simulink model "RTR_1st"  (R2020a)
settings: Solver=ode45  StartTime=0.0  StopTime=T  RelTol=1e-8
values from neighbouring files (symbols this model uses):
  g = 9.81    [TestingIkRTR.m]    (also in TestingScript.m; TestingScriptRTR.m)
  Kd1 = Kp1/10    (= 100)    [TestingIkRTR.m]    (also in TestingScript.m; TestingScriptRTR.m)
  Kp1 = 1000    [TestingIkRTR.m]    (also in TestingScript.m; TestingScriptRTR.m)
  l2 = 0.3    [TestingIkRTR.m]    (also in TestingScriptRTR.m)
  l3 = 0.2    [TestingIkRTR.m]    (also in TestingScriptRTR.m)
  m2 = 20    [TestingIkRTR.m]    (also in TestingScriptRTR.m)
  m3 = 20    [TestingIkRTR.m]    (also in TestingScriptRTR.m)
settings Model: Creator=ja  LastModifiedBy=ja

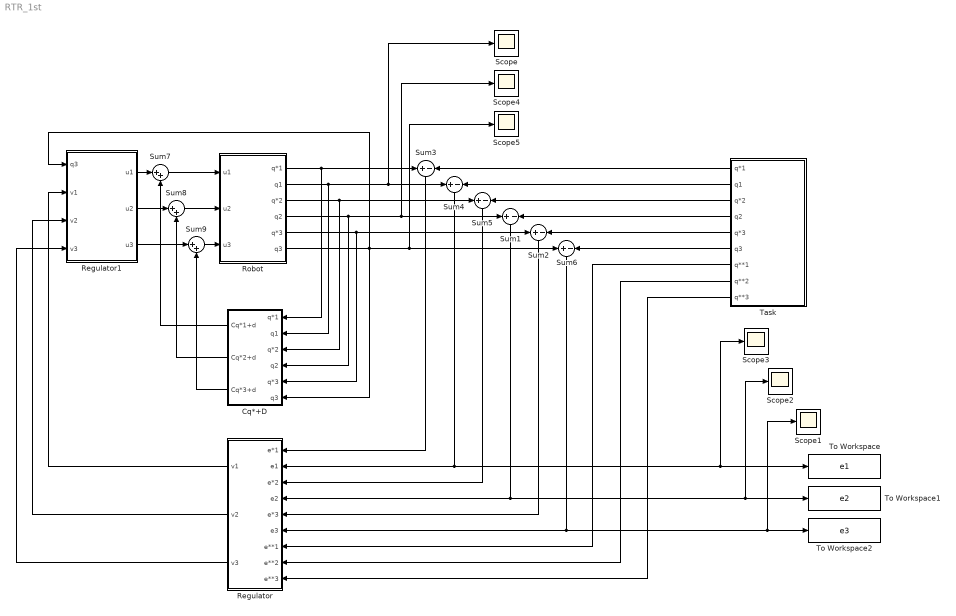
== system RTR_1st ==
  Cq*+D : Subsystem
  Regulator : Subsystem
  Regulator1 : Subsystem
  Robot : Subsystem
  Scope{,1..5} (6 alike) : Scope
  Sum{1..6} (6 alike) : Sum  Inputs=+-
  Sum7 : Sum  Inputs=|++
  Sum8 : Sum  Inputs=|++
  Sum9 : Sum  Inputs=|++
  Task : Subsystem
  To Workspace : ToWorkspace  VariableName=e1  SampleTime=-1
  To Workspace1 : ToWorkspace  VariableName=e2  SampleTime=-1
  To Workspace2 : ToWorkspace  VariableName=e3  SampleTime=-1
  wires:
  Robot/1(q*1) -> Cq*+D/1(q*1), Sum3/1
  Task/1(q*1) -> Sum3/2
  Robot/2(q1) -> Cq*+D/2(q1), Scope/1, Sum4/1
  Task/2(q1) -> Sum4/2
  Task/3(q*2) -> Sum5/2
  Robot/3(q*2) -> Cq*+D/3(q*2), Sum5/1
  Task/4(q2) -> Sum1/2
  Robot/4(q2) -> Cq*+D/4(q2), Scope4/1, Sum1/1
  Task/5(q*3) -> Sum2/2
  Robot/5(q*3) -> Cq*+D/5(q*3), Sum2/1
  Task/6(q3) -> Sum6/2
  Robot/6(q3) -> Regulator1/1(q3), Cq*+D/6(q3), Scope5/1, Sum6/1
  Sum3/1 -> Regulator/1(e*1)
  Sum4/1 -> Scope3/1, To Workspace/1, Regulator/2(e1)
  Sum5/1 -> Regulator/3(e*2)
  Sum1/1 -> Scope2/1, To Workspace1/1, Regulator/4(e2)
  Sum2/1 -> Regulator/5(e*3)
  Sum6/1 -> Scope1/1, To Workspace2/1, Regulator/6(e3)
  Regulator/1(" v1") -> Regulator1/2(v1)
  Regulator/2(v2) -> Regulator1/3(v2)
  Regulator/3(v3) -> Regulator1/4(v3)
  Sum7/1 -> Robot/1(u1)
  Regulator1/1(" u1") -> Sum7/1
  Regulator1/2(u2) -> Sum8/1
  Sum8/1 -> Robot/2(u2)
  Regulator1/3(u3) -> Sum9/1
  Sum9/1 -> Robot/3(u3)
  Cq*+D/1(" Cq*1+d") -> Sum7/2
  Cq*+D/2(Cq*2+d) -> Sum8/2
  Cq*+D/3(Cq*3+d) -> Sum9/2
  Task/7(q**1) -> Regulator/7(e**1)
  Task/8(q**2) -> Regulator/8(e**2)
  Task/9(q**3) -> Regulator/9(e**3)

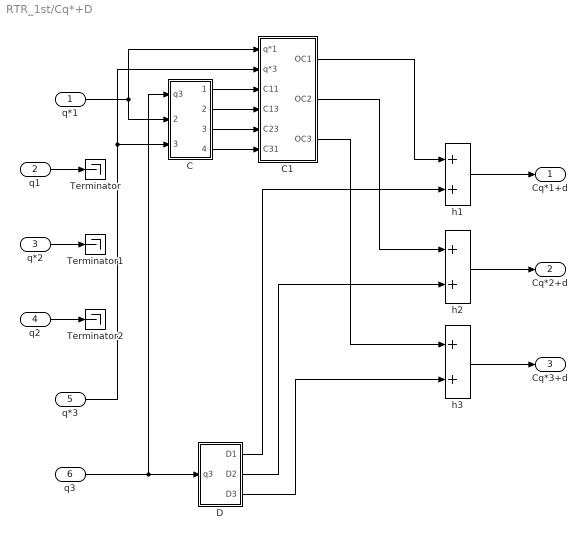
== system RTR_1st/Cq*+D ==
  q*1 : Inport
  q1 : Inport  Port=2
  q*2 : Inport  Port=3
  q2 : Inport  Port=4
  q*3 : Inport  Port=5
  q3 : Inport  Port=6
  C : Subsystem
  C1 : Subsystem
  D : Subsystem
  Terminator : Terminator
  Terminator1 : Terminator
  Terminator2 : Terminator
  h1 : Sum
  h2 : Sum
  h3 : Sum
  " Cq*1+d" : Outport
  Cq*2+d : Outport  Port=2
  Cq*3+d : Outport  Port=3
  wires:
  D/1(D1) -> h1/2
  D/2(D2) -> h2/2
  C1/2(OC2) -> h2/1
  D/3(D3) -> h3/2
  C/2(C13) -> C1/4(C13)
  C/1(C11) -> C1/3(C11)
  C/3(C23) -> C1/5(C23)
  C1/1(OC1) -> h1/1
  C/4(C31) -> C1/6(C31)
  C1/3(OC3) -> h3/1
  q3/1 -> C/1(q3), D/1(q3)
  h1/1 -> " Cq*1+d"/1
  h2/1 -> Cq*2+d/1
  h3/1 -> Cq*3+d/1
  q*1/1 -> C1/1(q*1), C/2(q*1)
  q*3/1 -> C/3(q*3), C1/2(q*3)
  q1/1 -> Terminator/1
  q*2/1 -> Terminator1/1
  q2/1 -> Terminator2/1

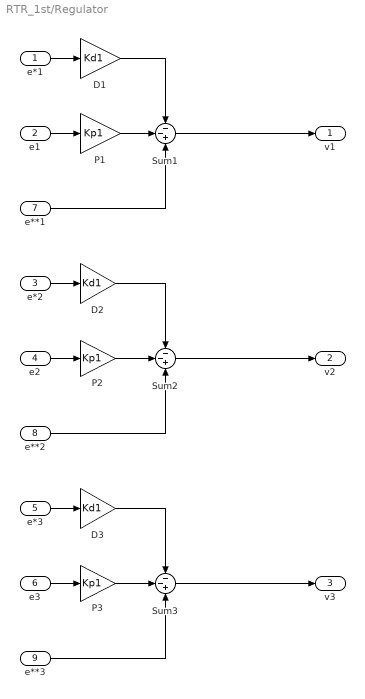
== system RTR_1st/Regulator ==
  e*1 : Inport
  e1 : Inport  Port=2
  e*2 : Inport  Port=3
  e2 : Inport  Port=4
  e*3 : Inport  Port=5
  e3 : Inport  Port=6
  e**1 : Inport  Port=7
  e**2 : Inport  Port=8
  e**3 : Inport  Port=9
  D1 : Gain  Gain=Kd1
  D2 : Gain  Gain=Kd1
  D3 : Gain  Gain=Kd1
  P1 : Gain  Gain=Kp1
  P2 : Gain  Gain=Kp1
  P3 : Gain  Gain=Kp1
  Sum1 : Sum  Inputs=--+
  Sum2 : Sum  Inputs=--+
  Sum3 : Sum  Inputs=--+
  " v1" : Outport
  v2 : Outport  Port=2
  v3 : Outport  Port=3
  wires:
  e2/1 -> P2/1
  Sum2/1 -> v2/1
  e*2/1 -> D2/1
  e1/1 -> P1/1
  Sum1/1 -> " v1"/1
  e*1/1 -> D1/1
  D1/1 -> Sum1/1
  P1/1 -> Sum1/2
  D2/1 -> Sum2/1
  P2/1 -> Sum2/2
  e*3/1 -> D3/1
  Sum3/1 -> v3/1
  P3/1 -> Sum3/2
  D3/1 -> Sum3/1
  e3/1 -> P3/1
  e**1/1 -> Sum1/3
  e**2/1 -> Sum2/3
  e**3/1 -> Sum3/3

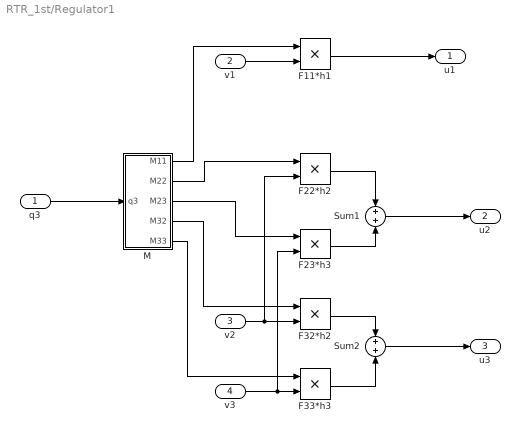
== system RTR_1st/Regulator1 ==
  q3 : Inport
  v1 : Inport  Port=2
  v2 : Inport  Port=3
  v3 : Inport  Port=4
  F11*h1 : Product
  F22*h2 : Product
  F23*h3 : Product
  F32*h2 : Product
  F33*h3 : Product
  M : Subsystem
  Sum1 : Sum
  Sum2 : Sum
  " u1" : Outport
  u2 : Outport  Port=2
  u3 : Outport  Port=3
  wires:
  q3/1 -> M/1(q3)
  F23*h3/1 -> Sum1/2
  F33*h3/1 -> Sum2/2
  F22*h2/1 -> Sum1/1
  F32*h2/1 -> Sum2/1
  v3/1 -> F23*h3/2, F33*h3/2
  v2/1 -> F22*h2/2, F32*h2/2
  v1/1 -> F11*h1/2
  M/1(M11) -> F11*h1/1
  M/2(M22) -> F22*h2/1
  M/3(M23) -> F23*h3/1
  M/4(M32) -> F32*h2/1
  M/5(M33) -> F33*h3/1
  F11*h1/1 -> " u1"/1
  Sum1/1 -> u2/1
  Sum2/1 -> u3/1

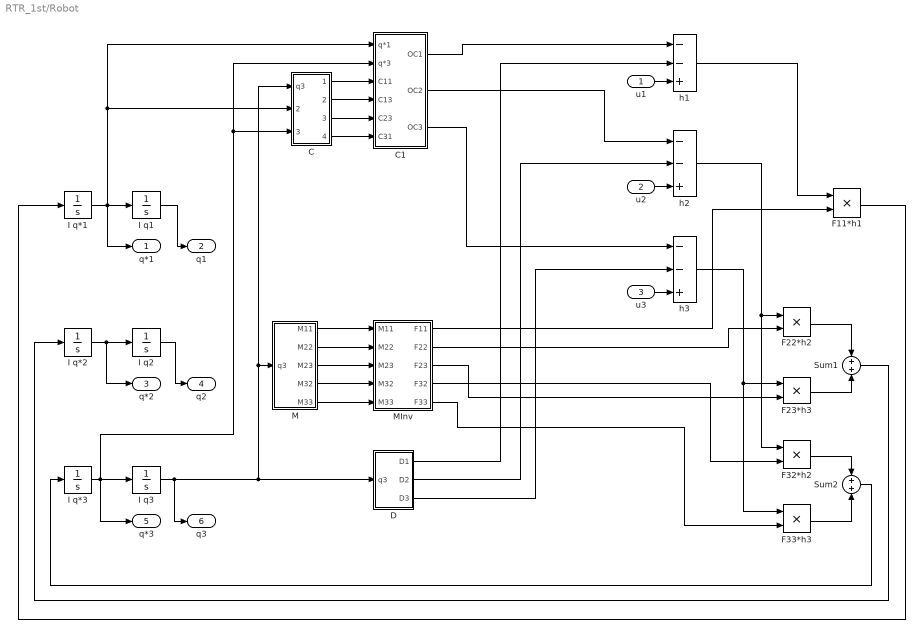
== system RTR_1st/Robot ==
  u1 : Inport
  u2 : Inport  Port=2
  u3 : Inport  Port=3
  C : Subsystem
  C1 : Subsystem
  D : Subsystem
  F11*h1 : Product
  F22*h2 : Product
  F23*h3 : Product
  F32*h2 : Product
  F33*h3 : Product
  I q*1 : Integrator
  I q*2 : Integrator
  I q*3 : Integrator
  I q1 : Integrator
  I q2 : Integrator
  I q3 : Integrator
  M : Subsystem
  MInv : MATLAB Function  TreatAsAtomicUnit=on
  Sum1 : Sum
  Sum2 : Sum
  h1 : Sum  Inputs=--+
  h2 : Sum  Inputs=--+
  h3 : Sum  Inputs=--+
  q*1 : Outport
  q1 : Outport  Port=2
  q*2 : Outport  Port=3
  q2 : Outport  Port=4
  q*3 : Outport  Port=5
  q3 : Outport  Port=6
  wires:
  I q2/1 -> q2/1
  F11*h1/1 -> I q*1/1
  I q*1/1 -> q*1/1, C1/1(q*1), C/2(q*1), I q1/1
  Sum1/1 -> I q*2/1
  I q1/1 -> q1/1
  F23*h3/1 -> Sum1/2
  I q*2/1 -> q*2/1, I q2/1
  F22*h2/1 -> Sum1/1
  u2/1 -> h2/3
  C/1(C11) -> C1/3(C11)
  C/2(C13) -> C1/4(C13)
  C/3(C23) -> C1/5(C23)
  C/4(C31) -> C1/6(C31)
  C1/1(OC1) -> h1/1
  F32*h2/1 -> Sum2/1
  F33*h3/1 -> Sum2/2
  Sum2/1 -> I q*3/1
  I q*3/1 -> C1/2(q*3), C/3(q*3), I q3/1, q*3/1
  I q3/1 -> q3/1, C/1(q3), M/1(q3), D/1(q3)
  u3/1 -> h3/3
  D/3(D3) -> h3/2
  D/2(D2) -> h2/2
  C1/2(OC2) -> h2/1
  C1/3(OC3) -> h3/1
  h2/1 -> F32*h2/1, F22*h2/1
  h3/1 -> F33*h3/1, F23*h3/1
  MInv/2(F22) -> F22*h2/2
  MInv/3(F23) -> F23*h3/2
  MInv/4(F32) -> F32*h2/2
  MInv/5(F33) -> F33*h3/2
  h1/1 -> F11*h1/1
  MInv/1(F11) -> F11*h1/2
  u1/1 -> h1/3
  D/1(D1) -> h1/2
  M/1(M11) -> MInv/1(M11)
  M/2(M22) -> MInv/2(M22)
  M/3(M23) -> MInv/3(M23)
  M/4(M32) -> MInv/4(M32)
  M/5(M33) -> MInv/5(M33)

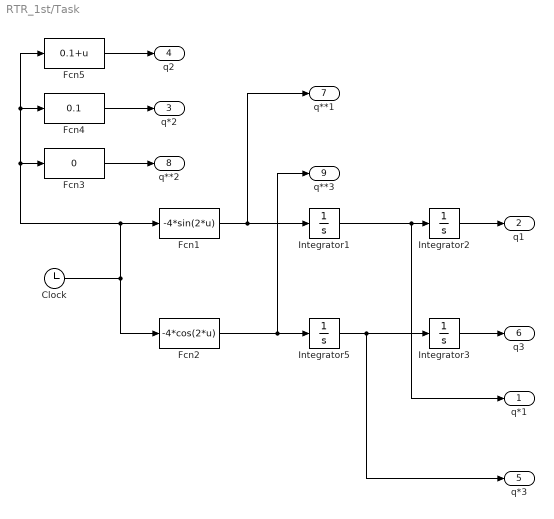
== system RTR_1st/Task ==
  Clock : Clock
  Fcn1 : Fcn  Expr=-4*sin(2*u)
  Fcn2 : Fcn  Expr=-4*cos(2*u)
  Fcn3 : Fcn  Expr=0
  Fcn4 : Fcn  Expr=0.1
  Fcn5 : Fcn  Expr=0.1+u
  Integrator1 : Integrator  InitialCondition=2
  Integrator2 : Integrator
  Integrator3 : Integrator  InitialCondition=1
  Integrator5 : Integrator
  q*1 : Outport
  q1 : Outport  Port=2
  q*2 : Outport  Port=3
  q2 : Outport  Port=4
  q*3 : Outport  Port=5
  q3 : Outport  Port=6
  q**1 : Outport  Port=7
  q**2 : Outport  Port=8
  q**3 : Outport  Port=9
  wires:
  Integrator2/1 -> q1/1
  Integrator3/1 -> q3/1
  Integrator1/1 -> q*1/1, Integrator2/1
  Integrator5/1 -> q*3/1, Integrator3/1
  Fcn1/1 -> Integrator1/1, q**1/1
  Fcn2/1 -> q**3/1, Integrator5/1
  Fcn3/1 -> q**2/1
  Fcn4/1 -> q*2/1
  Fcn5/1 -> q2/1
  Clock/1 -> Fcn5/1, Fcn4/1, Fcn3/1, Fcn1/1, Fcn2/1

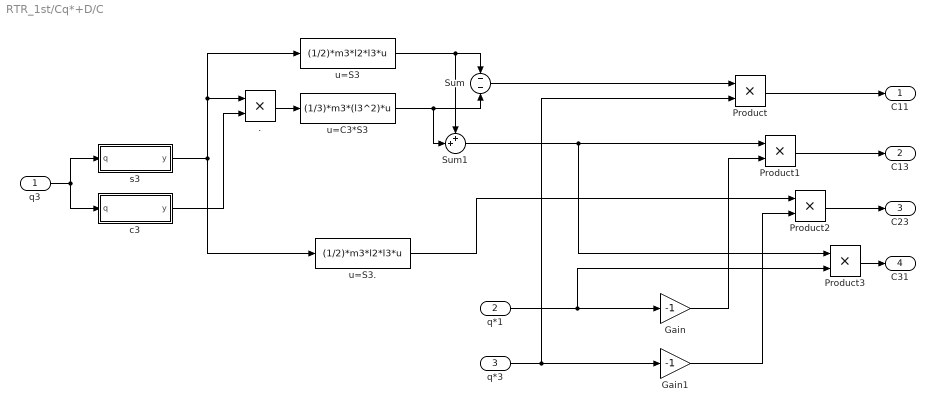
== system RTR_1st/Cq*+D/C ==
  q3 : Inport
  q*1 : Inport  Port=2
  q*3 : Inport  Port=3
  . : Product
  Gain : Gain  Gain=-1
  Gain1 : Gain  Gain=-1
  Product{,1..3} (4 alike) : Product
  Sum : Sum  Inputs=--
  Sum1 : Sum  Inputs=++|
  c3 : MATLAB Function  TreatAsAtomicUnit=on
  s3 : MATLAB Function  TreatAsAtomicUnit=on
  u=C3*S3 : Fcn  Expr=(1/3)*m3*(l3^2)*u
  u=S3 : Fcn  Expr=(1/2)*m3*l2*l3*u
  u=S3. : Fcn  Expr=(1/2)*m3*l2*l3*u
  C11 : Outport
  C13 : Outport  Port=2
  C23 : Outport  Port=3
  C31 : Outport  Port=4
  wires:
  q3/1 -> s3/1(q), c3/1(q)
  c3/1(y) -> ./2
  s3/1(y) -> u=S3./1, ./1, u=S3/1
  ./1 -> u=C3*S3/1
  u=C3*S3/1 -> Sum1/2, Sum/2
  u=S3/1 -> Sum1/1, Sum/1
  Gain1/1 -> Product2/2
  Product/1 -> C11/1
  Product2/1 -> C23/1
  Product1/1 -> C13/1
  Sum/1 -> Product/1
  q*1/1 -> Gain/1, Product3/2
  q*3/1 -> Gain1/1, Product/2
  Product3/1 -> C31/1
  Gain/1 -> Product1/2
  Sum1/1 -> Product1/1, Product3/1
  u=S3./1 -> Product2/1

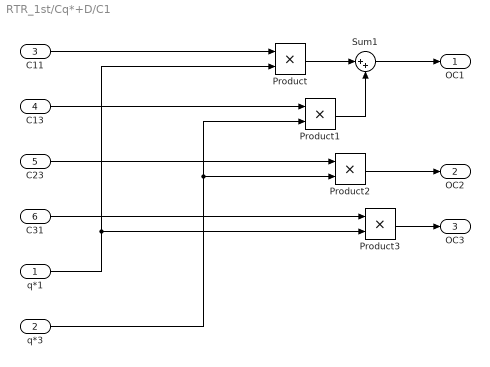
== system RTR_1st/Cq*+D/C1 ==
  q*1 : Inport
  q*3 : Inport  Port=2
  C11 : Inport  Port=3
  C13 : Inport  Port=4
  C23 : Inport  Port=5
  C31 : Inport  Port=6
  Product{,1..3} (4 alike) : Product
  Sum1 : Sum  Inputs=|++
  OC1 : Outport
  OC2 : Outport  Port=2
  OC3 : Outport  Port=3
  wires:
  C11/1 -> Product/1
  C13/1 -> Product1/1
  C23/1 -> Product2/1
  C31/1 -> Product3/1
  Product3/1 -> OC3/1
  Product2/1 -> OC2/1
  q*1/1 -> Product3/2, Product/2
  q*3/1 -> Product2/2, Product1/2
  Product/1 -> Sum1/1
  Sum1/1 -> OC1/1
  Product1/1 -> Sum1/2

== system RTR_1st/Cq*+D/D ==
  q3 : Inport
  . : Fcn  Expr=1/2*m3*l3*u
  Constant : Constant  Value=g
  Constant1 : Constant  Value=m3
  Constant2 : Constant  Value=m2
  Constant3 : Constant  Value=0
  Product : Product
  Product1 : Product
  Sum : Sum
  c3 : MATLAB Function  TreatAsAtomicUnit=on
  D1 : Outport
  D2 : Outport  Port=2
  D3 : Outport  Port=3
  wires:
  c3/1(y) -> ./1
  Sum/1 -> Product/1
  Constant/1 -> Product/2, Product1/1
  ./1 -> Product1/2
  Constant2/1 -> Sum/2
  Constant1/1 -> Sum/1
  q3/1 -> c3/1(q)
  Product/1 -> D2/1
  Product1/1 -> D3/1
  Constant3/1 -> D1/1

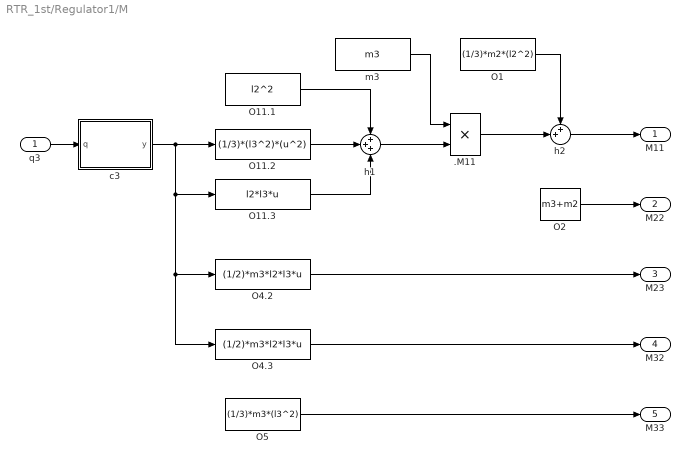
== system RTR_1st/Regulator1/M ==
  q3 : Inport
  .M11 : Product
  O1 : Constant  Value=(1/3)*m2*(l2^2)
  O11.1 : Constant  Value=l2^2
  O11.2 : Fcn  Expr=(1/3)*(l3^2)*(u^2)
  O11.3 : Fcn  Expr=l2*l3*u
  O2 : Constant  Value=m3+m2
  O4.2 : Fcn  Expr=(1/2)*m3*l2*l3*u
  O4.3 : Fcn  Expr=(1/2)*m3*l2*l3*u
  O5 : Constant  Value=(1/3)*m3*(l3^2)
  c3 : MATLAB Function  TreatAsAtomicUnit=on
  h1 : Sum  Inputs=+++
  h2 : Sum  Inputs=++|
  m3 : Constant  Value=m3
  M11 : Outport
  M22 : Outport  Port=2
  M23 : Outport  Port=3
  M32 : Outport  Port=4
  M33 : Outport  Port=5
  wires:
  O1/1 -> h2/1
  O11.3/1 -> h1/3
  m3/1 -> .M11/1
  h1/1 -> .M11/2
  .M11/1 -> h2/2
  O11.1/1 -> h1/1
  O11.2/1 -> h1/2
  h2/1 -> M11/1
  O2/1 -> M22/1
  O4.2/1 -> M23/1
  c3/1(y) -> O11.2/1, O4.3/1, O4.2/1, O11.3/1
  q3/1 -> c3/1(q)
  O5/1 -> M33/1
  O4.3/1 -> M32/1

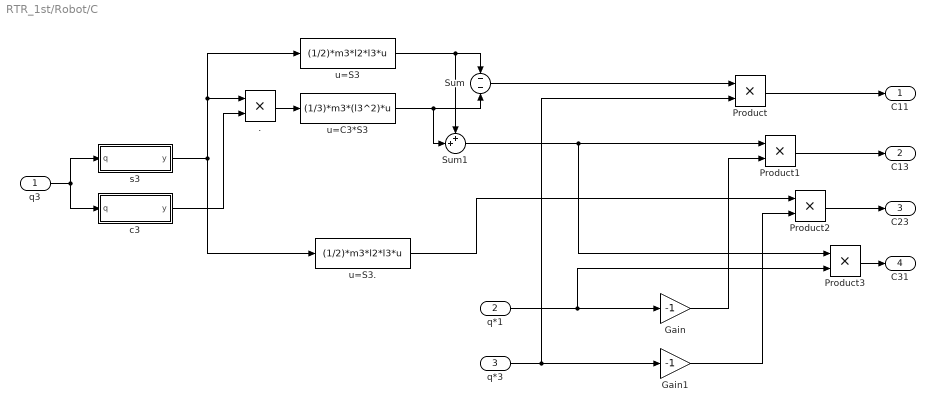
== system RTR_1st/Robot/C ==
  q3 : Inport
  q*1 : Inport  Port=2
  q*3 : Inport  Port=3
  . : Product
  Gain : Gain  Gain=-1
  Gain1 : Gain  Gain=-1
  Product{,1..3} (4 alike) : Product
  Sum : Sum  Inputs=--
  Sum1 : Sum  Inputs=++|
  c3 : MATLAB Function  TreatAsAtomicUnit=on
  s3 : MATLAB Function  TreatAsAtomicUnit=on
  u=C3*S3 : Fcn  Expr=(1/3)*m3*(l3^2)*u
  u=S3 : Fcn  Expr=(1/2)*m3*l2*l3*u
  u=S3. : Fcn  Expr=(1/2)*m3*l2*l3*u
  C11 : Outport
  C13 : Outport  Port=2
  C23 : Outport  Port=3
  C31 : Outport  Port=4
  wires:
  q3/1 -> s3/1(q), c3/1(q)
  c3/1(y) -> ./2
  s3/1(y) -> u=S3./1, ./1, u=S3/1
  ./1 -> u=C3*S3/1
  u=C3*S3/1 -> Sum1/2, Sum/2
  u=S3/1 -> Sum1/1, Sum/1
  Gain1/1 -> Product2/2
  Product/1 -> C11/1
  Product2/1 -> C23/1
  Product1/1 -> C13/1
  Sum/1 -> Product/1
  q*1/1 -> Gain/1, Product3/2
  q*3/1 -> Gain1/1, Product/2
  Product3/1 -> C31/1
  Gain/1 -> Product1/2
  Sum1/1 -> Product1/1, Product3/1
  u=S3./1 -> Product2/1

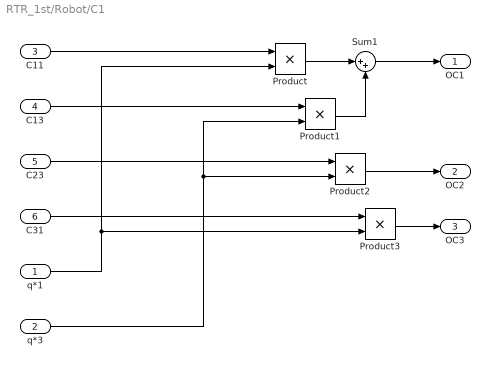
== system RTR_1st/Robot/C1 ==
  q*1 : Inport
  q*3 : Inport  Port=2
  C11 : Inport  Port=3
  C13 : Inport  Port=4
  C23 : Inport  Port=5
  C31 : Inport  Port=6
  Product{,1..3} (4 alike) : Product
  Sum1 : Sum  Inputs=|++
  OC1 : Outport
  OC2 : Outport  Port=2
  OC3 : Outport  Port=3
  wires:
  C11/1 -> Product/1
  C13/1 -> Product1/1
  C23/1 -> Product2/1
  C31/1 -> Product3/1
  Product3/1 -> OC3/1
  Product2/1 -> OC2/1
  q*1/1 -> Product3/2, Product/2
  q*3/1 -> Product2/2, Product1/2
  Product/1 -> Sum1/1
  Sum1/1 -> OC1/1
  Product1/1 -> Sum1/2

== system RTR_1st/Robot/D ==
  q3 : Inport
  . : Fcn  Expr=1/2*m3*l3*u
  Constant : Constant  Value=g
  Constant1 : Constant  Value=m3
  Constant2 : Constant  Value=m2
  Constant3 : Constant  Value=0
  Product : Product
  Product1 : Product
  Sum : Sum
  c3 : MATLAB Function  TreatAsAtomicUnit=on
  D1 : Outport
  D2 : Outport  Port=2
  D3 : Outport  Port=3
  wires:
  c3/1(y) -> ./1
  Sum/1 -> Product/1
  Constant/1 -> Product/2, Product1/1
  ./1 -> Product1/2
  Constant2/1 -> Sum/2
  Constant1/1 -> Sum/1
  q3/1 -> c3/1(q)
  Product/1 -> D2/1
  Product1/1 -> D3/1
  Constant3/1 -> D1/1

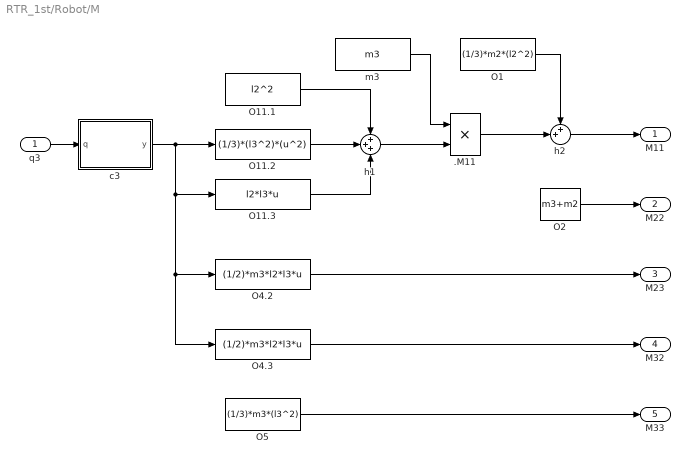
== system RTR_1st/Robot/M ==
  q3 : Inport
  .M11 : Product
  O1 : Constant  Value=(1/3)*m2*(l2^2)
  O11.1 : Constant  Value=l2^2
  O11.2 : Fcn  Expr=(1/3)*(l3^2)*(u^2)
  O11.3 : Fcn  Expr=l2*l3*u
  O2 : Constant  Value=m3+m2
  O4.2 : Fcn  Expr=(1/2)*m3*l2*l3*u
  O4.3 : Fcn  Expr=(1/2)*m3*l2*l3*u
  O5 : Constant  Value=(1/3)*m3*(l3^2)
  c3 : MATLAB Function  TreatAsAtomicUnit=on
  h1 : Sum  Inputs=+++
  h2 : Sum  Inputs=++|
  m3 : Constant  Value=m3
  M11 : Outport
  M22 : Outport  Port=2
  M23 : Outport  Port=3
  M32 : Outport  Port=4
  M33 : Outport  Port=5
  wires:
  O1/1 -> h2/1
  O11.3/1 -> h1/3
  m3/1 -> .M11/1
  h1/1 -> .M11/2
  .M11/1 -> h2/2
  O11.1/1 -> h1/1
  O11.2/1 -> h1/2
  h2/1 -> M11/1
  O2/1 -> M22/1
  O4.2/1 -> M23/1
  c3/1(y) -> O11.2/1, O4.3/1, O4.2/1, O11.3/1
  q3/1 -> c3/1(q)
  O5/1 -> M33/1
  O4.3/1 -> M32/1

== matlab function RTR_1st/Robot/M/c3 ==
  data: q input; y output
function y = c(q)

y = cos(q);

== matlab function RTR_1st/Robot/C/c3 ==
  data: q input; y output
function y = c(q)

y = cos(q);

== matlab function RTR_1st/Robot/D/c3 ==
  data: q input; y output
function y = c(q)

y = cos(q);

== matlab function RTR_1st/Cq*+D/C/c3 ==
  data: q input; y output
function y = c(q)

y = cos(q);

== matlab function RTR_1st/Robot/C/s3 ==
  data: q input; y output
function y = s(q)

y = sin(q);

== matlab function RTR_1st/Robot/MInv ==
  data: M11 input; M22 input; F11 output; F22 output; M23 input; M32 input; F23 output; F32 output; M33 input; F33 output
function [F11, F22, F23, F32, F33] = c(M11, M22, M23, M32, M33)

M = [M11 0 0; 0 M22 M23; 0 M32 M33];
F = inv(M);

F11 = F(1);
F22 = F(5);
F23 = F(6);
F32 = F(8);
F33 = F(9);

== matlab function RTR_1st/Cq*+D/C/s3 ==
  data: q input; y output
function y = s(q)

y = sin(q);

== matlab function RTR_1st/Cq*+D/D/c3 ==
  data: q input; y output
function y = c(q)

y = cos(q);

== matlab function RTR_1st/Regulator1/M/c3 ==
  data: q input; y output
function y = c(q)

y = cos(q);
